simulink model "nine"  (R2020b)
settings: Solver=VariableStepAuto  StartTime=0.0  StopTime=10.0  RelTol=1e-3
settings Model: Creator=Dell  LastModifiedBy=Dell

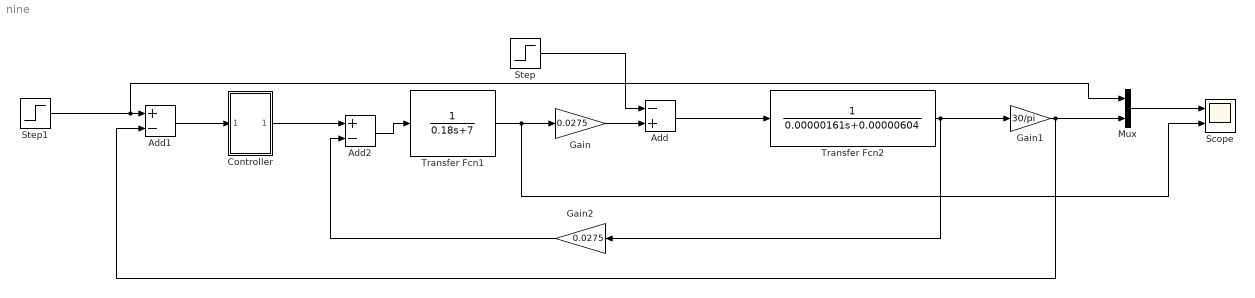
== system nine ==
  Add : Sum  Inputs=-+
  Add1 : Sum  Inputs=+-
  Add2 : Sum  Inputs=+-
  Controller : Subsystem
  Gain : Gain  Gain=0.0275
  Gain1 : Gain  Gain=30/pi
  Gain2 : Gain  Gain=0.0275
  Mux : Mux  Inputs=2
  Scope : Scope  NumInputPorts=2
  Step : Step  SampleTime=0
  Step1 : Step  SampleTime=0
  Transfer Fcn1 : TransferFcn  Denominator=[0.18 7]
  Transfer Fcn2 : TransferFcn  Denominator=[0.00000161 0.00000604]
  wires:
  Add1/1 -> Controller/1(In1)
  Controller/1(Out1) -> Add2/1
  Gain2/1 -> Add2/2
  Mux/1 -> Scope/1
  Add2/1 -> Transfer Fcn1/1
  Step1/1 -> Mux/1, Add1/1
  Step/1 -> Add/1
  Transfer Fcn1/1 -> Scope/2, Gain/1
  Add/1 -> Transfer Fcn2/1
  Gain1/1 -> Add1/2, Mux/2
  Transfer Fcn2/1 -> Gain2/1, Gain1/1
  Gain/1 -> Add/2

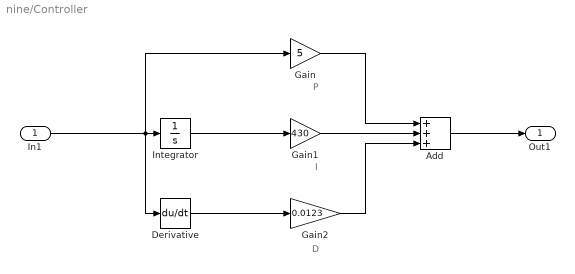
== system nine/Controller ==
  note: D
  note: I
  note: P
  In1 : Inport
  Add : Sum  Inputs=+++
  Derivative : Derivative
  Gain : Gain  Gain=5
  Gain1 : Gain  Gain=430
  Gain2 : Gain  Gain=0.0123
  Integrator : Integrator
  Out1 : Outport
  wires:
  Gain2/1 -> Add/3
  In1/1 -> Derivative/1, Gain/1, Integrator/1
  Integrator/1 -> Gain1/1
  Derivative/1 -> Gain2/1
  Gain1/1 -> Add/2
  Gain/1 -> Add/1
  Add/1 -> Out1/1
